simulink model "cartpole"  (R2023b)
settings: Solver=FixedStepAuto  StartTime=0.0  StopTime=20  FixedStep=0.01  RelTol=1e-3
settings Model: Creator=gomes  LastModifiedBy=gomes
settings SolverCC: AlgebraicLoopSolver=TrustRegion
settings DebuggingCC: UnconnectedInputMsg=warning  UnconnectedOutputMsg=warning  UnconnectedLineMsg=warning
settings ModelReferenceCC: EnableRefExpFcnMdlSchedulingChecks=on
settings RTWCC: DLArmComputeVersion=19.05

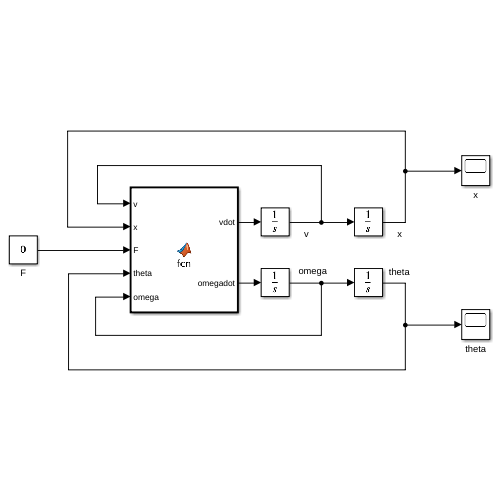
[thumbnail: Simulink's stored preview of the top-level diagram]
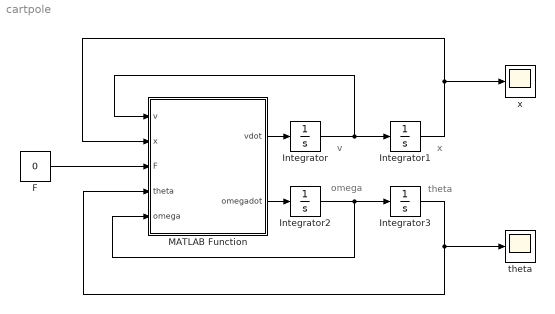
== system cartpole ==
  note: x
  note: v
  note: omega
  note: theta
  F : Constant  Value=0
  Integrator{,1..3} (4 alike) : Integrator
  MATLAB Function : MATLAB Function  TreatAsAtomicUnit=on
  theta : Scope
  x : Scope
  wires:
  Integrator2/1 -> MATLAB Function/5(omega), Integrator3/1
  Integrator/1 -> MATLAB Function/1(v), Integrator1/1
  Integrator1/1 -> x/1, MATLAB Function/2(x)
  Integrator3/1 -> theta/1, MATLAB Function/4(theta)
  MATLAB Function/1(vdot) -> Integrator/1
  MATLAB Function/2(omegadot) -> Integrator2/1
  F/1 -> MATLAB Function/3(F)

== matlab function cartpole/MATLAB Function ==
  data: v input; x input; vdot output; omegadot output; F input; theta input; omega input
function [vdot,omegadot] = fcn(v,x,F,theta,omega)

m = 0.2;
M = 0.4;
l = 0.3;
g = 9.8;

btheta = 0.2;
bx = 0.2;

ct = cos(theta);
st = sin(theta);

A = [ct , 4*l/3 ; M+m  ,m*l*ct];
b = [st*g-btheta*omega ; m*l*st*omega^2+F-bx*v];

sol = A\b;

vdot     = sol(1);
omegadot = sol(2);
